simulink library "satellite_control_lib"  (R2015b)
settings: Solver=ode45  StartTime=0.0  StopTime=10.0  RelTol=1e-3
undefined symbols (not defined in the file or in its folder): DiscIntNeverNeededParam
libraries: aerolibutil x5, vrlib x3, dspmtrx3 x1
settings Model: Creator=DNikolaev  LastModifiedBy=DNikolaev
settings DataIOCC: SaveFormat=Array
settings DebuggingCC: UnderspecifiedInitializationDetection=Classic  MergeDetectMultiDrivingBlocksExec=none  SolverPrmCheckMsg=warning
settings HardwareCC: ProdBitPerPointer=32  ProdLargestAtomicFloat=None  ProdIntDivRoundTo=Undefined  ProdEndianess=Unspecified  ProdWordSize=32  ProdHWDeviceType=32-bit Generic
settings GRTTargetCC: GeneratePreprocessorConditionals=Disable all
settings ConfigComp: CovModelRefEnable=Off

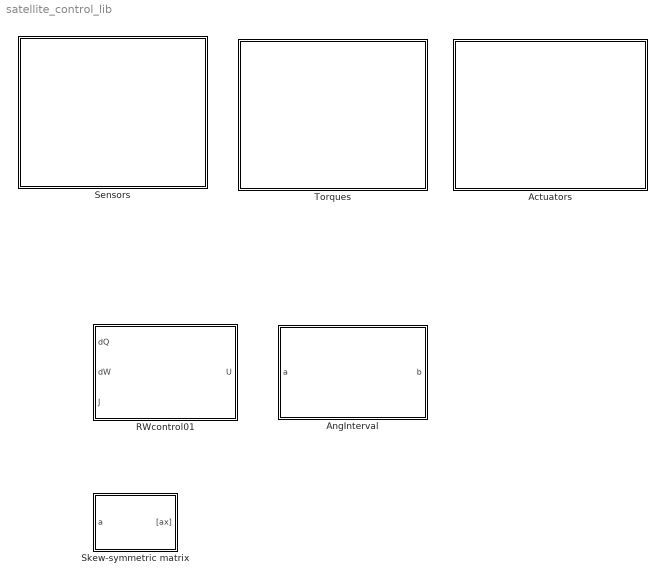
== system satellite_control_lib ==
  Actuators : Subsystem
      mask Display: text(0.5,0.5, 'Actuators','hor','center')
  AngInterval : MATLAB Function  TreatAsAtomicUnit=on
  RWcontrol01 : Subsystem  mask{Kq=1, Kw=1}
      mask DialogControl DescTextVar Prompt: Control algorithm U=J*(Kq*dQ+Kw*dW)
      mask Display:
      | disp('U=J(Kq*f(dQ)+Kw*dW)')
      | port_label('input',1,'dQ')
      | port_label('input',2,'dW')
      | port_label('input',3,'J')
      | port_label('output',1,'U')
  Sensors : Subsystem
      mask Display: text(0.5,0.5, 'Sensors','hor','center')
  Skew-symmetric matrix : Subsystem
      mask DialogControl DescTextVar Prompt: Create 3x3 skew-symmetric matrix from vector
      mask Display:
      | port_label('input', 1, 'A')
      | port_label('output', 1, '[Ax]')
  Torques : Subsystem
      mask Display: text(0.5,0.5, 'Torques','hor','center')

== system satellite_control_lib/Actuators ==
  Magnetic Coils : Subsystem  mask{MagnMomentMax=50}
      mask prompts: MagnMomentMax "Maximum magnetic moment, Am2"
  Reaction Wheels 4-pyramid configuration : Subsystem  VariantControl=Variant  mask{Hrwmax=20, Trwmax=0.1, delta=55, gamma=45, sampleTime=0.1}
      mask prompts: Hrwmax "Maximum kinetic moment, Nms"; Trwmax "Maximum torque, Nm"; delta "Delta angle, deg"; gamma "Gamma angle, deg"; sampleTime "Sample Time"
      mask Display:
      | port_label('input', 1, 'Trwreq_b')
      | port_label('output', 1, 'Trwreq_p')
      | port_label('output', 2, 'Hrw_p')

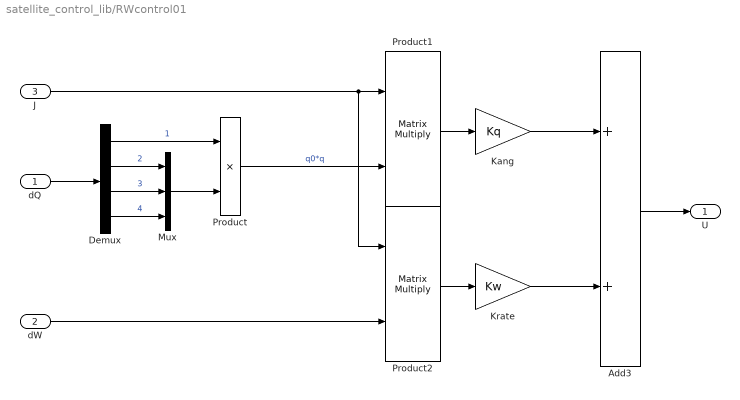
== system satellite_control_lib/RWcontrol01 ==
  dQ : Inport
  dW : Inport  Port=2
  J : Inport  Port=3
  Add3 : Sum
  Demux : Demux
  Kang : Gain  Gain=Kq  SampleTime=Kw
  Krate : Gain  Gain=Kw
  Mux : Mux  Inputs=3
  Product : Product
  Product1 : Product  Multiplication=Matrix(*)
  Product2 : Product  Multiplication=Matrix(*)
  U : Outport
  wires:
  dQ/1 -> Demux/1
  Demux/1 -> Product/1  "1"
  Demux/2 -> Mux/1  "2"
  Demux/3 -> Mux/2  "3"
  Demux/4 -> Mux/3  "4"
  Mux/1 -> Product/2
  J/1 -> Product2/1, Product1/1
  dW/1 -> Product2/2
  Product1/1 -> Kang/1
  Product2/1 -> Krate/1
  Krate/1 -> Add3/2
  Kang/1 -> Add3/1
  Add3/1 -> U/1
  Product/1 -> Product1/2  "q0*q"

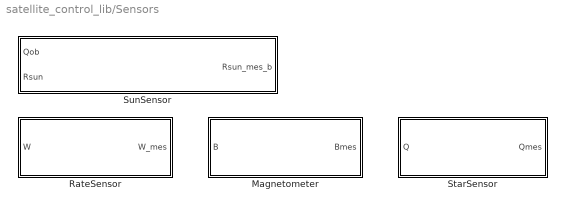
== system satellite_control_lib/Sensors ==
  Magnetometer : Subsystem  mask{S=[0 0 0;0 0 0;0 0 0], bias=0, sigma2=0, seed=0, outputSampleTime=0.1}
      mask prompts: S "Scale factor"; sigma2 "Variance"; outputSampleTime "Output sample time"
      mask Display: text(0.5,0.5,'B^{mes}=(I_{3}+S)B^{true}+\beta^{true}+\eta_\nu','hor','center','texmode','on')
  RateSensor : Subsystem  mask{S=[0 0 0;0 0 0;0 0 0], sigma2_b=0, seed_b=[0 0 0], sigma2_n=0, seed=[0 0 0], rateSensorSamleTime=0.1}
      mask prompts: S "Scale factor"; sigma2_b "Bias variance (sigma2)"; seed_b "Seed for bias"; sigma2_n "Variance (sigma2)"; rateSensorSamleTime "Output samle time"
      mask Display: text(0.5,0.5,'\omega=(I_3+S)\omega^{true}+\beta^{true}+\eta_\nu','hor','center','texmode','on')
  StarSensor : Subsystem  mask{sigma2=[0 0 0], seed=[0 0 0], outputSamleTime=0.1}
      mask prompts: sigma2 "Variance"; outputSamleTime "Output sample time"
      mask Display: text(0.5,0.5,'Q_{j bmes}=Q_{j b} \circ Q_{noise}','hor','center','texmode','on')
  SunSensor : Subsystem  mask{sigma2=[0 0 0], seed=[0 0 0], outputSampleTime=0.1}
      mask prompts: sigma2 "Variance"; outputSampleTime "Output samle time"
      mask Display:
      | text(0.5,0.5,'R_{sun mes b} = quatrot (Q_{o b} \circ Q_{noise}, R_{sun o} )','hor','center','texmode','on')
      | port_label('input', 1, 'Qob')
      | port_label('input', 2, 'Rsun_o')

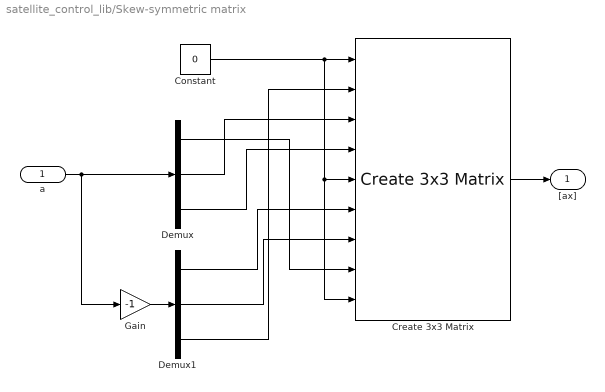
== system satellite_control_lib/Skew-symmetric matrix ==
  a : Inport
  Constant : Constant  Value=0
  Create 3x3 Matrix : aerolibutil/Create 3x3 Matrix
  Demux : Demux  Outputs=3
  Demux1 : Demux  Outputs=3
  Gain : Gain  Gain=-1
  "[ax]" : Outport
  wires:
  a/1 -> Gain/1, Demux/1
  Constant/1 -> Create 3x3 Matrix/5, Create 3x3 Matrix/9, Create 3x3 Matrix/1
  Gain/1 -> Demux1/1
  Demux1/3 -> Create 3x3 Matrix/2
  Demux/2 -> Create 3x3 Matrix/3
  Demux/3 -> Create 3x3 Matrix/4
  Demux1/1 -> Create 3x3 Matrix/6
  Demux1/2 -> Create 3x3 Matrix/7
  Demux/1 -> Create 3x3 Matrix/8
  Create 3x3 Matrix/1 -> "[ax]"/1

== system satellite_control_lib/Torques ==
  Tgrav : Subsystem
  Tmagn : Subsystem
  Trw : Subsystem  mask{delta=55, gamma=45}
      mask prompts: delta "Delta angle, deg"; gamma "Gamma angle, deg"

== system satellite_control_lib/Actuators/Magnetic Coils ==
  magnMomentReq : Inport
  Rate Transition : RateTransition  OutPortSampleTime=0.001
  Saturation : Saturate  UpperLimit=MagnMomentMax  LowerLimit=-MagnMomentMax
  magnMoment : Outport
  wires:
  magnMomentReq/1 -> Rate Transition/1
  Rate Transition/1 -> Saturation/1
  Saturation/1 -> magnMoment/1

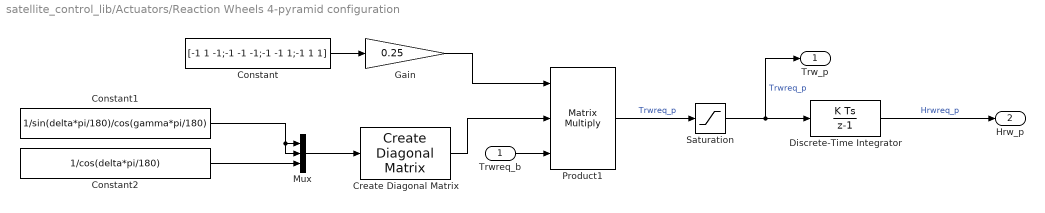
== system satellite_control_lib/Actuators/Reaction Wheels 4-pyramid configuration ==
  Trwreq_b : Inport
  Constant : Constant  Value=[-1 1 -1;-1 -1 -1;-1 -1 1;-1 1 1]
  Constant1 : Constant  Value=1/sin(delta*pi/180)/cos(gamma*pi/180)
  Constant2 : Constant  Value=1/cos(delta*pi/180)
  Create Diagonal Matrix : dspmtrx3/Create Diagonal Matrix
  Discrete-Time Integrator : DiscreteIntegrator  InitialConditionSetting=State (most efficient)  SampleTime=sampleTime  LimitOutput=on  UpperSaturationLimit=Hrwmax  LowerSaturationLimit=-Hrwmax  ICPrevOutput=DiscIntNeverNeededParam  ICPrevScaledInput=DiscIntNeverNeededParam
  Gain : Gain  Gain=0.25
  Mux : Mux  Inputs=3
  Product1 : Product  Inputs=3  Multiplication=Matrix(*)
  Saturation : Saturate  UpperLimit=Trwmax  LowerLimit=-Trwmax
  Trw_p : Outport
  Hrw_p : Outport  Port=2
  wires:
  Saturation/1 -> Trw_p/1, Discrete-Time Integrator/1  "Trwreq_p"
  Discrete-Time Integrator/1 -> Hrw_p/1  "Hrwreq_p"
  Constant/1 -> Gain/1
  Gain/1 -> Product1/1
  Create Diagonal Matrix/1 -> Product1/2
  Constant1/1 -> Mux/2, Mux/1
  Mux/1 -> Create Diagonal Matrix/1
  Constant2/1 -> Mux/3
  Trwreq_b/1 -> Product1/3
  Product1/1 -> Saturation/1  "Trwreq_p"

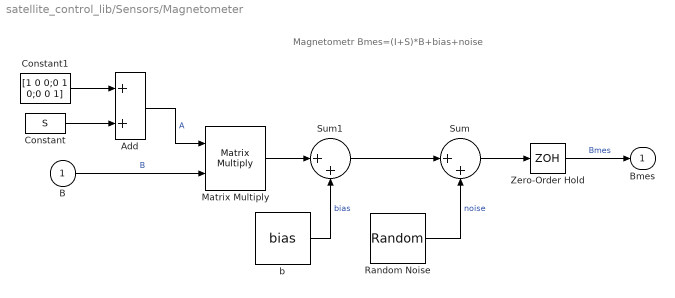
== system satellite_control_lib/Sensors/Magnetometer ==
  note: Magnetometr
      | Bmes=(I+S)*B+bias+noise
  B : Inport
  Add : Sum
  Constant : Constant  Value=S
  Constant1 : Constant  Value=[1 0 0;0 1 0;0 0 1]  VectorParams1D=off
  Matrix Multiply : Product  Multiplication=Matrix(*)
  Random Noise : RandomNumber  Variance=sigma2  Seed=seed
  Sum : Sum  Inputs=|++
  Sum1 : Sum  Inputs=|++
  Zero-Order Hold : ZeroOrderHold  SampleTime=outputSampleTime
  b : Constant  Value=bias
  Bmes : Outport
  wires:
  Random Noise/1 -> Sum/2  "noise"
  Sum/1 -> Zero-Order Hold/1
  Add/1 -> Matrix Multiply/1  "A"
  Matrix Multiply/1 -> Sum1/1
  B/1 -> Matrix Multiply/2  "B"
  b/1 -> Sum1/2  "bias"
  Sum1/1 -> Sum/1
  Zero-Order Hold/1 -> Bmes/1  "Bmes"
  Constant1/1 -> Add/1
  Constant/1 -> Add/2

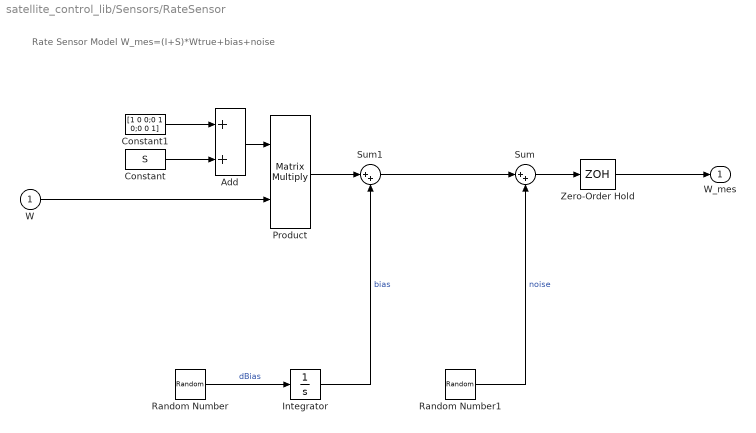
== system satellite_control_lib/Sensors/RateSensor ==
  note: Rate Sensor Model
      | W_mes=(I+S)*Wtrue+bias+noise
  W : Inport
  Add : Sum
  Constant : Constant  Value=S
  Constant1 : Constant  Value=[1 0 0;0 1 0;0 0 1]  VectorParams1D=off
  Integrator : Integrator
  Product : Product  Multiplication=Matrix(*)
  Random Number : RandomNumber  Mean=[0 0 0]  Variance=sigma2_b  Seed=seed_b
  Random Number1 : RandomNumber  Variance=sigma2_n  Seed=seed(2)
  Sum : Sum  Inputs=|++
  Sum1 : Sum  Inputs=|++
  Zero-Order Hold : ZeroOrderHold  SampleTime=rateSensorSamleTime
  W_mes : Outport
  wires:
  W/1 -> Product/2
  Sum/1 -> Zero-Order Hold/1
  Sum1/1 -> Sum/1
  Constant1/1 -> Add/1
  Constant/1 -> Add/2
  Add/1 -> Product/1
  Product/1 -> Sum1/1
  Random Number1/1 -> Sum/2  "noise"
  Integrator/1 -> Sum1/2  "bias"
  Random Number/1 -> Integrator/1  "dBias"
  Zero-Order Hold/1 -> W_mes/1

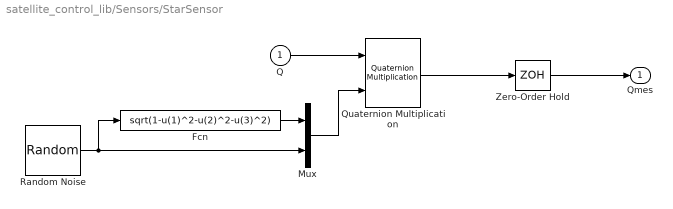
== system satellite_control_lib/Sensors/StarSensor ==
  Q : Inport
  Fcn : Fcn  Expr=sqrt(1-u(1)^2-u(2)^2-u(3)^2)
  Mux : Mux  Inputs=2
  Quaternion Multiplication : aerolibutil/Quaternion Multiplication
  Random Noise : RandomNumber  Mean=[0 0 0]  Variance=sigma2  Seed=seed
  Zero-Order Hold : ZeroOrderHold  SampleTime=outputSamleTime
  Qmes : Outport
  wires:
  Zero-Order Hold/1 -> Qmes/1
  Q/1 -> Quaternion Multiplication/1
  Mux/1 -> Quaternion Multiplication/2
  Quaternion Multiplication/1 -> Zero-Order Hold/1
  Random Noise/1 -> Mux/2, Fcn/1
  Fcn/1 -> Mux/1

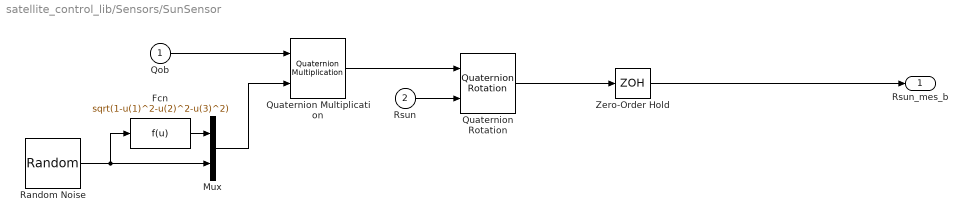
== system satellite_control_lib/Sensors/SunSensor ==
  Qob : Inport
  Rsun : Inport  Port=2
  Fcn : Fcn  Expr=sqrt(1-u(1)^2-u(2)^2-u(3)^2)
  Mux : Mux  Inputs=2
  Quaternion Multiplication : aerolibutil/Quaternion Multiplication
  Quaternion Rotation : aerolibutil/Quaternion Rotation
  Random Noise : RandomNumber  Mean=[0 0 0]  Variance=sigma2  Seed=seed
  Zero-Order Hold : ZeroOrderHold  SampleTime=outputSampleTime
  Rsun_mes_b : Outport
  wires:
  Rsun/1 -> Quaternion Rotation/2
  Quaternion Multiplication/1 -> Quaternion Rotation/1
  Quaternion Rotation/1 -> Zero-Order Hold/1
  Mux/1 -> Quaternion Multiplication/2
  Qob/1 -> Quaternion Multiplication/1
  Zero-Order Hold/1 -> Rsun_mes_b/1
  Random Noise/1 -> Fcn/1, Mux/2
  Fcn/1 -> Mux/1

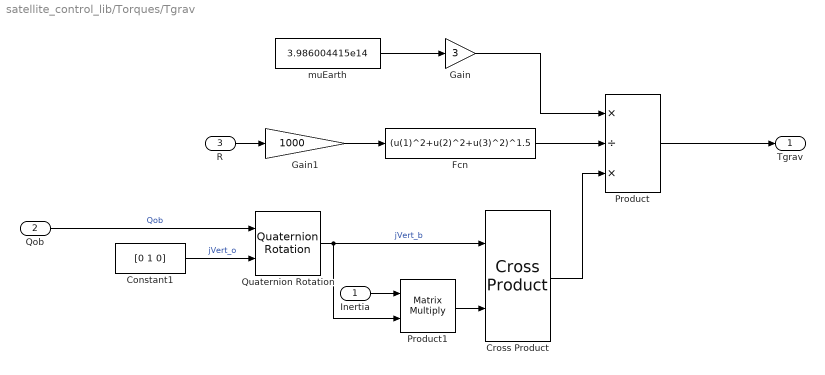
== system satellite_control_lib/Torques/Tgrav ==
  Inertia : Inport
  Qob : Inport  Port=2
  R : Inport  Port=3
  Constant1 : Constant  Value=[0 1 0]
  Cross Product : vrlib/Utilities/Cross Product
  Fcn : Fcn  Expr=(u(1)^2+u(2)^2+u(3)^2)^1.5
  Gain : Gain  Gain=3
  Gain1 : Gain  Gain=1000
  Product : Product  Inputs=*/*
  Product1 : Product  Multiplication=Matrix(*)
  Quaternion Rotation : aerolibutil/Quaternion Rotation
  muEarth : Constant  Value=3.986004415e14
  Tgrav : Outport
  wires:
  Constant1/1 -> Quaternion Rotation/2  "jVert_o"
  Qob/1 -> Quaternion Rotation/1  "Qob"
  Quaternion Rotation/1 -> Product1/2, Cross Product/1  "jVert_b"
  Inertia/1 -> Product1/1
  Product1/1 -> Cross Product/2
  muEarth/1 -> Gain/1
  Gain/1 -> Product/1
  Cross Product/1 -> Product/3
  R/1 -> Gain1/1
  Fcn/1 -> Product/2
  Product/1 -> Tgrav/1
  Gain1/1 -> Fcn/1

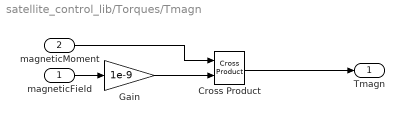
== system satellite_control_lib/Torques/Tmagn ==
  magneticField : Inport
  magneticMoment : Inport  Port=2
  Cross Product : vrlib/Utilities/Cross Product
  Gain : Gain  Gain=1e-9
  Tmagn : Outport
  wires:
  magneticField/1 -> Gain/1
  Gain/1 -> Cross Product/2
  magneticMoment/1 -> Cross Product/1
  Cross Product/1 -> Tmagn/1

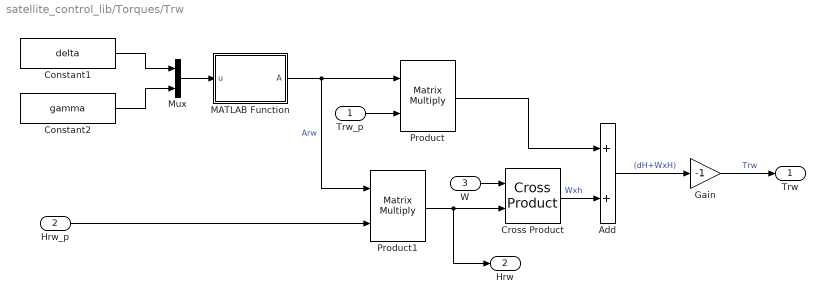
== system satellite_control_lib/Torques/Trw ==
  Trw_p : Inport
  Hrw_p : Inport  Port=2
  W : Inport  Port=3
  Add : Sum
  Constant1 : Constant  Value=delta
  Constant2 : Constant  Value=gamma
  Cross Product : vrlib/Utilities/Cross Product
  Gain : Gain  Gain=-1
  MATLAB Function : MATLAB Function  TreatAsAtomicUnit=on
  Mux : Mux  Inputs=2
  Product : Product  Multiplication=Matrix(*)
  Product1 : Product  Multiplication=Matrix(*)
  Trw : Outport
  Hrw : Outport  Port=2
  wires:
  W/1 -> Cross Product/1
  Cross Product/1 -> Add/2  "Wxh"
  Add/1 -> Gain/1  "(dH+WxH)"
  Gain/1 -> Trw/1  "Trw"
  Constant1/1 -> Mux/1
  Constant2/1 -> Mux/2
  Mux/1 -> MATLAB Function/1(u)
  MATLAB Function/1(A) -> Product/1, Product1/1  "Arw"
  Trw_p/1 -> Product/2
  Product/1 -> Add/1
  Hrw_p/1 -> Product1/2
  Product1/1 -> Hrw/1, Cross Product/2

== matlab function satellite_control_lib/Torques/Trw/MATLAB Function ==
  data: u input; A output
function A = fcn(u)
delta = u(1)*pi/180;
gamma = u(2)*pi/180;

sd=sin(delta);
cd=cos(delta);
sg=sin(gamma);
cg=cos(gamma);
A=[-sd*cg -sd*cg -sd*cg -sd*cg;
      sd*sg -sd*sg -sd*sg  sd*sg;
      -cd    -cd     cd     cd];

== matlab function satellite_control_lib/AngInterval ==
  data: a input; b output
function b = AngInterval(a)
% Переводит любой угол в радианах в отрезок [-pi;pi]
b=a-fix((a+sign(a)*pi)/(2*pi))*2*pi;
